simulink model "project_model_part4_watermarking_detector2"  (R2020a)
settings: Solver=VariableStepAuto  StartTime=0.0  StopTime=130  RelTol=1e-3
undefined symbols (not defined in the file or in its folder): Discrete, Time
libraries: ctrlSharedLib x1
settings Model: Creator=Admin  LastModifiedBy=Shreya
settings DataIOCC: ReturnWorkspaceOutputs=off
settings DebuggingCC: ArithmeticOperatorsInVariantConditions=warning
settings SFSimCC: SimUseLocalCustomCode=off  CustomCodeUndefinedFunction=UseInterfaceOnly
settings RTWCC: RTWUseLocalCustomCode=off

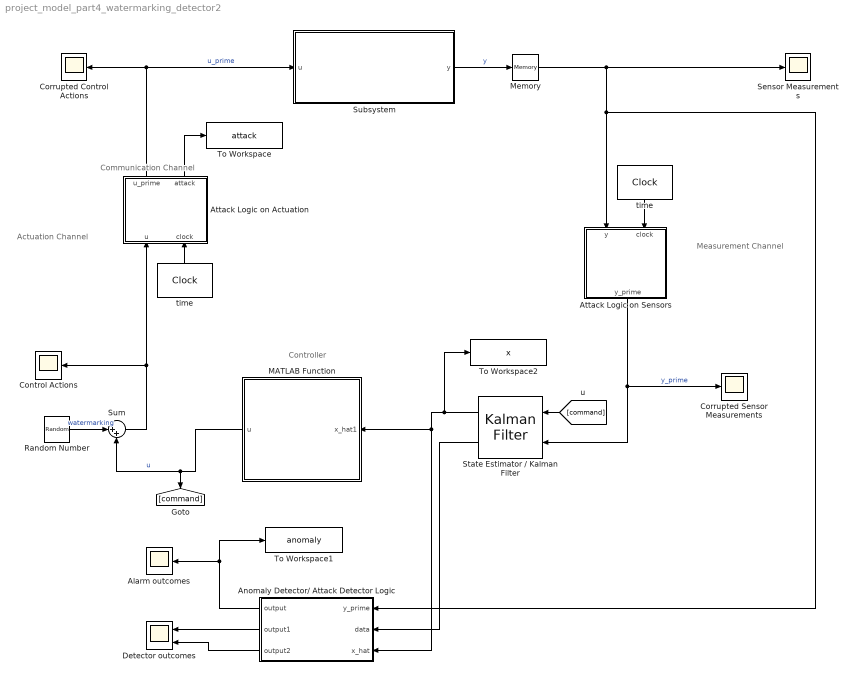
== system project_model_part4_watermarking_detector2 ==
  note: Controller
  note: Communication Channel
  note: Measurement Channel
  note: Actuation Channel
  Alarm outcomes : Scope
  Anomaly Detector/ Attack Detector Logic : MATLAB Function  TreatAsAtomicUnit=on
  Attack Logic on Actuation : MATLAB Function  TreatAsAtomicUnit=on
  Attack Logic on Sensors : MATLAB Function  TreatAsAtomicUnit=on
  Control Actions : Scope
  Corrupted Control Actions : Scope
  Corrupted Sensor Measurements : Scope
  Detector outcomes : Scope  NumInputPorts=2
  MATLAB Function : MATLAB Function  TreatAsAtomicUnit=on
  Memory : Memory  InitialCondition=[0,0]  InheritSampleTime=on
  Random Number : RandomNumber  Variance=0.00001  Seed=[0,0]  SampleTime=0.1
  "Sensor Measurements " : Scope
  State Estimator / Kalman Filter : ctrlSharedLib/Kalman Filter  TimeDomain=Discrete-Time  UseCurrentEstimator=on  ModelSource=Individual A, B, C, D matrices  ModelSourceVariable=sys  A="[1.0000    0.0001   -0.0010;0.5747    1.0000   -0.0003;0.0162    0.0000    1.0000]"  B="[0.1   -0.2; -0.0536    0.0332;0.1955   -0.5294];"  C=[1 0 0;0 1 0]  D=[0 0;0 0]  NumberOfStates=2  NumberOfInputs=2  NumberOfOutputs=2  InitialEstimateSource=Dialog  X0=[0;0;0]  P0=10  UseK=off  UseGH=off  NumberOfProcessNoiseInputs=2  G=1  TimeInvariantG=on  H=0  TimeInvariantH=on  Q=0.00001*eye(3)  TimeInvariantQ=on  R=0.00008*eye(2)  TimeInvariantR=on  N=0  TimeInvariantN=on  AddInputPort=on  AddEnablePort=off  OutputEstimatedY=off  OutputP=on  Ts=-1
  Subsystem : Subsystem
  Sum : Sum  Inputs=|++  RndMeth=Convergent
  To Workspace : ToWorkspace  VariableName=attack  SaveFormat=Timeseries  SampleTime=0.1
  To Workspace1 : ToWorkspace  VariableName=anomaly  SaveFormat=Timeseries  SampleTime=0.1
  To Workspace2 : ToWorkspace  VariableName=x  SaveFormat=Timeseries  SampleTime=0.1
  time : DigitalClock  SampleTime=0.1
  "time " : DigitalClock  SampleTime=0.1
  wires:
  "time "/1 -> Attack Logic on Sensors/2(clock)
  Attack Logic on Sensors/1(y_prime) -> State Estimator / Kalman Filter/2, Corrupted Sensor Measurements/1  "y_prime"
  time/1 -> Attack Logic on Actuation/2(clock)
  Attack Logic on Actuation/1(u_prime) -> Corrupted Control Actions/1, Subsystem/1(u)  "u_prime"
  [command] -> State Estimator / Kalman Filter/1
  State Estimator / Kalman Filter/1 -> To Workspace2/1, MATLAB Function/1(x_hat1), Anomaly Detector/ Attack Detector Logic/3(x_hat)
  Sum/1 -> Attack Logic on Actuation/1(u), Control Actions/1
  MATLAB Function/1(u) -> Sum/2, [command]  "u"
  State Estimator / Kalman Filter/2 -> Anomaly Detector/ Attack Detector Logic/2(data)
  Random Number/1 -> Sum/1  "watermarking"
  Anomaly Detector/ Attack Detector Logic/1(output) -> To Workspace1/1, Alarm outcomes/1
  Subsystem/1(y) -> Memory/1  "y"
  Memory/1 -> "Sensor Measurements "/1, Anomaly Detector/ Attack Detector Logic/1(y_prime), Attack Logic on Sensors/1(y)
  Attack Logic on Actuation/2(attack) -> To Workspace/1
  Anomaly Detector/ Attack Detector Logic/2(output1) -> Detector outcomes/1
  Anomaly Detector/ Attack Detector Logic/3(output2) -> Detector outcomes/2

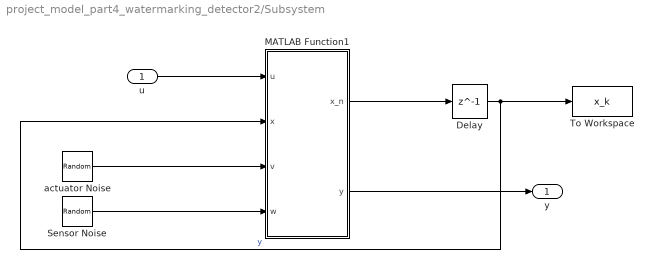
== system project_model_part4_watermarking_detector2/Subsystem ==
  u : Inport
  Delay : Delay  DelayLength=1  InitialCondition=[0 0.1 0.2]
  MATLAB Function1 : MATLAB Function  TreatAsAtomicUnit=on
  Sensor Noise : RandomNumber  Mean=[0 0]  Variance=[0.00008 0.00008]  Seed=[randi(100) randi(100)]
  To Workspace : ToWorkspace  VariableName=x_k  SaveFormat=Timeseries  SampleTime=-1
  actuator Noise : RandomNumber  Mean=[0 0 0]  Variance=[0.00001 0.00001 0.00001]  Seed=[randi(100) randi(100) randi(100)]
  y : Outport  VectorParamsAs1DForOutWhenUnconnected=off
  wires:
  u/1 -> MATLAB Function1/1(u)
  MATLAB Function1/1(x_n) -> Delay/1
  MATLAB Function1/2(y) -> y/1
  Sensor Noise/1 -> MATLAB Function1/4(w)
  actuator Noise/1 -> MATLAB Function1/3(v)
  Delay/1 -> To Workspace/1, MATLAB Function1/2(x)  "y"

== matlab function project_model_part4_watermarking_detector2/Attack Logic on Sensors ==
  data: y input; y_prime output; clock input
function y_prime = fcn(y,clock)
% this function should contain the attacker action on the sensor
% measurements
%Replay Attacl logic
y_prime = y;
persistent i
persistent j
persistent n
if isempty(i)
    i = 1;
end
if isempty(j)
    j = 1;
end
if isempty(n)
    n = zeros(200,2); 
end
if clock >= 80 && clock < 100
    % Recored data between 80 to 100
    n(i,:) = transpose(y);
    i = i+1;  
elseif clock >= 100 && clock < 120
    % input Recored data between 100 to 120
    y_prime = transpose(n(j,:));
    j = j+1;
else
    y_prime = y;
end
end

== matlab function project_model_part4_watermarking_detector2/MATLAB Function ==
  data: x_hat1 input; u output
function u  = Controller(x_hat1)
%two tanks model 
    

%controller gain
K = [17.1291   -1.1789   -6.5335; -0.1248   -2.9385   -2.5082];
u = -K*(x_hat1);

== matlab function project_model_part4_watermarking_detector2/Attack Logic on Actuation ==
  data: u input; u_prime output; clock input; attack output
function [u_prime,attack] = fcn(u,clock)
% this function should contain the attacker action on the control inputs
%Attck logic on Actuation Channel
if clock < 100
    u_prime = u + transpose([0,0]);
    attack = 0;
elseif clock >= 100 && clock < 120
    u_prime = u + transpose([-0.05 ,-0.05]);
    attack = 1;
else 
    u_prime = u + transpose([0,0]);
    attack =0;
end
end

== matlab function project_model_part4_watermarking_detector2/Anomaly Detector// Attack Detector Logic ==
  data: output output; y_prime input; data input; x_hat input; output1 output; output2 output
function [output ,output1 ,output2] = Detector(y_prime, data, x_hat)
% this function should contain the detection strategy

% CUSUM detector logic
C = [1 0 0; 0 1 0];
R = 0.00008*eye(2);
%Here P is error covarience.
P = data;
sigma = (C * P * (transpose(C))) + R;
r = y_prime - (C * x_hat);
% Choosen Distance Measure but it is possible to drive CUSUM with any other distance measure
z = transpose(r) * (inv(sigma) * r);
%Here b is 'bias parameter'. For the tightest detection b is similar to P(state estimater error Covarience)
%Since z >= 0, the bias parameter b prevents the inherent growth due to the sum of nonnegative number.
%bias b must be selected properly based on the properties of the distance measure.
b = 2;
persistent s;
if isempty(s)
    %intially Cumulative sum is zero
    s = 0;
end
%Here beta is threshold value. 
%Once the bias is chosen, the threshold bita must be selected to fulfill a required false alarm rate.
beta = 13.5;
if s <= beta
    s = max([0,s + z - b]);
    output = 0;
else
    s = 0;
    output = 1;
end
output1 = s;
output2 = beta;
end

== matlab function project_model_part4_watermarking_detector2/Subsystem/MATLAB Function1 ==
  data: x_n output; u input; y output; x input; v input; w input
function [x_n, y] = fcn(u, x, v, w)

A=[1.0000    0.0001   -0.0010;0.5747    1.0000   -0.0003;0.0162    0.0000    1.0000];
B = [0.1   -0.2; -0.0536    0.0332;0.1955   -0.5294];

C=[1 0 0;0 1 0];
D=[0 0;0 0];


x_n = A*x + B*u + v;
y = C*x + D*u + w;
